simulink model "pitch"  (R2014b)
settings: Solver=ode1  StartTime=0.0  StopTime=10  FixedStep=0.1  RelTol=1e-3
values from neighbouring files (symbols this model uses):
  delta = pi/16    (= 0.196349540849)    [pitch_main.m]
  J = 15    [pitch_main.m]
  k_2 = 5    [pitch_main.m]
  k_3 = 1    [pitch_main.m]
  k_4 = 1    [pitch_main.m]
settings Model: Creator=rende_000  LastModifiedBy=rende_000

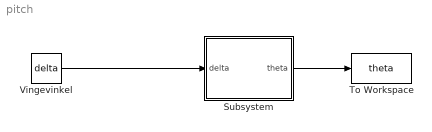
== system pitch ==
  Subsystem : Subsystem
  To Workspace : ToWorkspace  VariableName=theta  SaveFormat=Timeseries  SampleTime=-1
  Vingevinkel : Constant  Value=delta
  wires:
  Vingevinkel/1 -> Subsystem/1(delta)
  Subsystem/1(theta) -> To Workspace/1

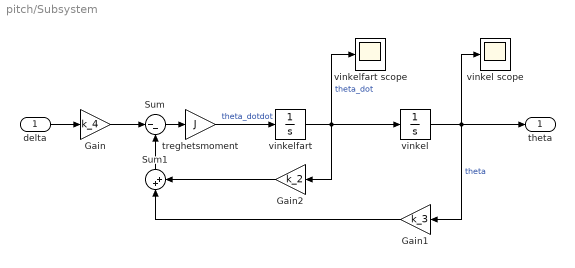
== system pitch/Subsystem ==
  delta : Inport
  Gain : Gain  Gain=k_4
  Gain1 : Gain  Gain=k_3
  Gain2 : Gain  Gain=k_2
  Sum : Sum  Inputs=|--
  Sum1 : Sum  Inputs=|++
  treghetsmoment : Gain  Gain=J
  vinkel : Integrator
  vinkel scope : Scope
  vinkelfart : Integrator
  vinkelfart scope : Scope
  theta : Outport
  wires:
  Sum/1 -> treghetsmoment/1
  Sum1/1 -> Sum/2
  treghetsmoment/1 -> vinkelfart/1  "theta_dotdot"
  delta/1 -> Gain/1
  Gain/1 -> Sum/1
  Gain2/1 -> Sum1/2
  Gain1/1 -> Sum1/1
  vinkelfart/1 -> Gain2/1, vinkelfart scope/1, vinkel/1  "theta_dot"
  vinkel/1 -> theta/1, vinkel scope/1, Gain1/1  "theta"
